simulink model "vtol_roll_kin_lin"  (R2021a)
settings: Solver=VariableStepAuto  StartTime=0.0  StopTime=100  RelTol=1e-3
undefined symbols (not defined in the file or in its folder): Ckf, disturbance_on, Klqr, noise_on, sys, sysKF, u1e, Vwind_ll, Vwind_ul
libraries: aerolibwind2 x1
settings Model: Creator=Tomo  LastModifiedBy=Tomo

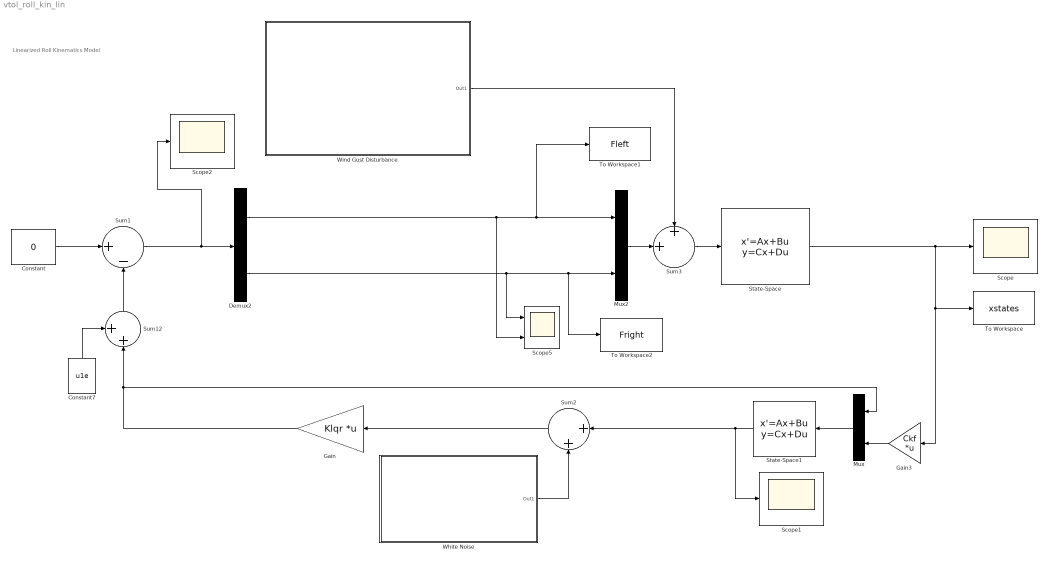
== system vtol_roll_kin_lin ==
  note: Linearized Roll Kinematics Model
  Constant : Constant  Value=0
  Constant7 : Constant  Value=u1e
  Demux2 : Demux  Outputs=2
  Gain : Gain  Gain=Klqr  Multiplication=Matrix(K*u)
  Gain3 : Gain  Gain=Ckf  Multiplication=Matrix(K*u)
  Mux : Mux  Inputs=2
  Mux2 : Mux  Inputs=2
  Scope : Scope
  Scope1 : Scope
  Scope2 : Scope
  Scope5 : Scope  NumInputPorts=2
  State-Space : StateSpace  A=sys.A  B=sys.B  C=sys.C  D=sys.D  InitialCondition=0
  State-Space1 : StateSpace  A=sysKF.A  B=sysKF.B  C=sysKF.C  D=sysKF.D  InitialCondition=0
  Sum1 : Sum  Inputs=|+-
  Sum12 : Sum  Inputs=++|
  Sum2 : Sum  Inputs=|++
  Sum3 : Sum  Inputs=++|
  To Workspace : ToWorkspace  VariableName=xstates  SaveFormat=Structure With Time  SampleTime=-1
  To Workspace1 : ToWorkspace  VariableName=Fleft  SaveFormat=Structure With Time  SampleTime=-1
  To Workspace2 : ToWorkspace  VariableName=Fright  SaveFormat=Structure With Time  SampleTime=-1
  White Noise : Subsystem
  Wind Gust Disturbance : Subsystem
  wires:
  Mux/1 -> State-Space1/1
  State-Space1/1 -> Scope1/1, Sum2/1
  Sum2/1 -> Gain/1
  White Noise/1(Out1) -> Sum2/2
  Sum1/1 -> Scope2/1, Demux2/1
  Sum3/1 -> State-Space/1
  Wind Gust Disturbance/1(Out1) -> Sum3/1
  Constant/1 -> Sum1/1
  Mux2/1 -> Sum3/2
  Demux2/1 -> Scope5/2, Mux2/1, To Workspace1/1
  Demux2/2 -> Scope5/1, Mux2/2, To Workspace2/1
  State-Space/1 -> To Workspace/1, Gain3/1, Scope/1
  Gain3/1 -> Mux/2
  Gain/1 -> Sum12/2, Mux/1
  Sum12/1 -> Sum1/2
  Constant7/1 -> Sum12/1

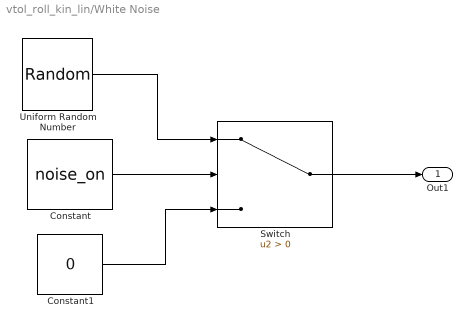
== system vtol_roll_kin_lin/White Noise ==
  Constant : Constant  Value=noise_on
  Constant1 : Constant  Value=0
  Switch : Switch  Criteria=u2 > Threshold
  Uniform Random Number : UniformRandomNumber  SampleTime=0.1
  Out1 : Outport
  wires:
  Constant/1 -> Switch/2
  Constant1/1 -> Switch/3
  Uniform Random Number/1 -> Switch/1
  Switch/1 -> Out1/1

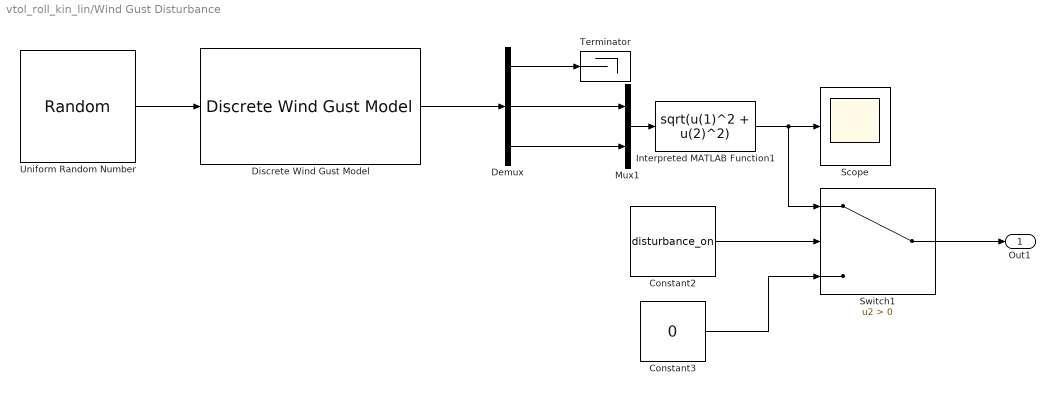
== system vtol_roll_kin_lin/Wind Gust Disturbance ==
  Constant2 : Constant  Value=disturbance_on
  Constant3 : Constant  Value=0
  Demux : Demux  Outputs=3
  Discrete Wind Gust Model : aerolibwind2/Discrete Wind Gust Model  units=Metric (MKS)  Gx=off  Gy=on  Gz=on  t_0=6  d_m=[120 120 80]  v_m=[23 23 23]
  Interpreted MATLAB Function1 : MATLABFcn  MATLABFcn=sqrt(u(1)^2 + u(2)^2)
  Mux1 : Mux  Inputs=2
  Scope : Scope
  Switch1 : Switch  Criteria=u2 > Threshold
  Terminator : Terminator
  Uniform Random Number : UniformRandomNumber  Minimum=Vwind_ll  Maximum=Vwind_ul  Seed=1  SampleTime=0.65
  Out1 : Outport
  wires:
  Demux/1 -> Terminator/1
  Discrete Wind Gust Model/1 -> Demux/1
  Uniform Random Number/1 -> Discrete Wind Gust Model/1
  Constant2/1 -> Switch1/2
  Constant3/1 -> Switch1/3
  Switch1/1 -> Out1/1
  Mux1/1 -> Interpreted MATLAB Function1/1
  Demux/2 -> Mux1/1
  Demux/3 -> Mux1/2
  Interpreted MATLAB Function1/1 -> Scope/1, Switch1/1
